simulink model "bit10counter"  (R2020a)
settings: Solver=VariableStepAuto  StartTime=0.0  StopTime=10.0  RelTol=1e-3
libraries: simulink_extras x10
settings Model: Creator=kishan  LastModifiedBy=kishan

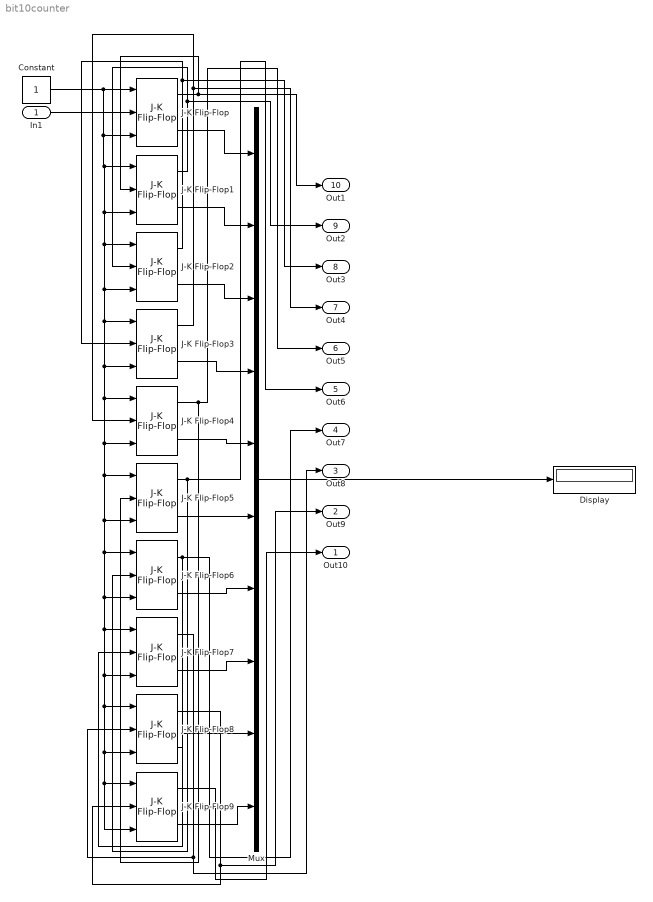
== system bit10counter ==
  In1 : Inport
  Constant : Constant
  Display : Display
  J-K Flip-Flop{,1..9} (10 alike) : simulink_extras/Flip Flops/J-K Flip-Flop  initial_condition=0
  Mux : Mux  Inputs=10
  Out10 : Outport
  Out9 : Outport  Port=2
  Out8 : Outport  Port=3
  Out7 : Outport  Port=4
  Out6 : Outport  Port=5
  Out5 : Outport  Port=6
  Out4 : Outport  Port=7
  Out3 : Outport  Port=8
  Out2 : Outport  Port=9
  Out1 : Outport  Port=10
  wires:
  Constant/1 -> J-K Flip-Flop9/3, J-K Flip-Flop9/1, J-K Flip-Flop8/3, J-K Flip-Flop8/1, J-K Flip-Flop7/3, J-K Flip-Flop7/1, J-K Flip-Flop6/3, J-K Flip-Flop6/1, J-K Flip-Flop5/3, J-K Flip-Flop5/1, J-K Flip-Flop4/3, J-K Flip-Flop4/1, J-K Flip-Flop3/3, J-K Flip-Flop3/1, J-K Flip-Flop2/3, J-K Flip-Flop2/1, J-K Flip-Flop1/3, J-K Flip-Flop1/1, J-K Flip-Flop/3, J-K Flip-Flop/1
  J-K Flip-Flop/1 -> Out1/1, J-K Flip-Flop1/2
  J-K Flip-Flop1/1 -> Out2/1, J-K Flip-Flop2/2
  J-K Flip-Flop2/1 -> Out3/1, J-K Flip-Flop3/2
  J-K Flip-Flop3/1 -> Out4/1, J-K Flip-Flop4/2
  J-K Flip-Flop4/1 -> Out5/1, J-K Flip-Flop5/2
  J-K Flip-Flop5/1 -> Out6/1, J-K Flip-Flop6/2
  J-K Flip-Flop6/1 -> Out7/1, J-K Flip-Flop7/2
  J-K Flip-Flop7/1 -> Out8/1, J-K Flip-Flop8/2
  J-K Flip-Flop8/1 -> Out9/1, J-K Flip-Flop9/2
  J-K Flip-Flop8/2 -> Mux/9
  J-K Flip-Flop9/2 -> Mux/10
  J-K Flip-Flop7/2 -> Mux/8
  J-K Flip-Flop6/2 -> Mux/7
  J-K Flip-Flop5/2 -> Mux/6
  J-K Flip-Flop4/2 -> Mux/5
  J-K Flip-Flop3/2 -> Mux/4
  J-K Flip-Flop2/2 -> Mux/3
  J-K Flip-Flop1/2 -> Mux/2
  J-K Flip-Flop/2 -> Mux/1
  Mux/1 -> Display/1
  In1/1 -> J-K Flip-Flop/2
  J-K Flip-Flop9/1 -> Out10/1
